simulink subsystem "Stewart_Platform"  (R2019b)
settings: Solver=VariableStepAuto  StartTime=0.0  StopTime=10.0  RelTol=1e-3
settings Model: Creator=thomas  LastModifiedBy=thomas

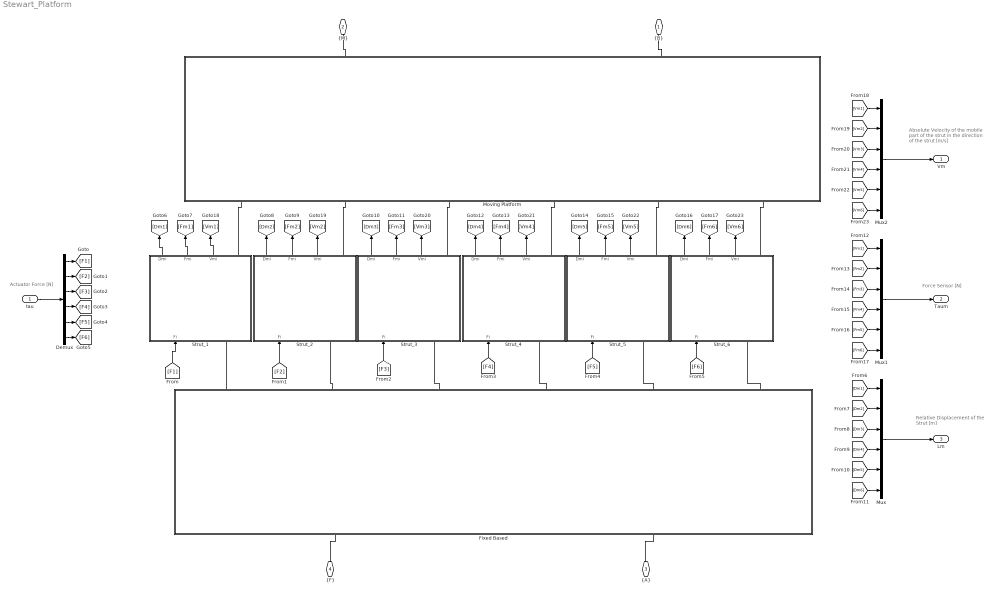
== system Stewart_Platform ==
  note: Force Sensor [N]
  note: Relative Displacement
      | of the Strut [m]
  note: Absolute Velocity of the
      | mobile part of the strut in
      | the direction of the strut [m/s]
  note: Actuator Force [N]
  tau : Inport
  Demux : Demux  Outputs=6
  Fixed Based : Subsystem  ReferencedSubsystem=Fixed_Based
  Moving Platform : Subsystem  ReferencedSubsystem=Mobile_Platform
  Mux : Mux  Inputs=6
  Mux1 : Mux  Inputs=6
  Mux2 : Mux  Inputs=6
  Strut_1 : Subsystem
      mask init:
      | i=1;
  Strut_2 : Subsystem
      mask init:
      | i=2;
  Strut_3 : Subsystem
      mask init:
      | i=3;
  Strut_4 : Subsystem
      mask init:
      | i=4;
  Strut_5 : Subsystem
      mask init:
      | i=5;
  Strut_6 : Subsystem
      mask init:
      | i=6;
  "{B}" : PMIOPort  Side=Right
  "{M}" : PMIOPort  Port=2  Side=Right
  "{A}" : PMIOPort  Port=3  Side=Left
  "{F}" : PMIOPort  Port=4  Side=Left
  Vm : Outport
  Taum : Outport  Port=2
  Lm : Outport  Port=3
  wires:
  [Vm3] -> Mux2/3
  [F3] -> Strut_3/1(Fi)
  [F4] -> Strut_4/1(Fi)
  Strut_5/1(Dmi) -> [Dm5]
  [F1] -> Strut_1/1(Fi)
  Strut_1/2(Fmi) -> [Fm1]
  Demux/5 -> [F5]
  Demux/1 -> [F1]
  Demux/6 -> [F6]
  [Fm2] -> Mux1/2
  Strut_3/1(Dmi) -> [Dm3]
  Demux/3 -> [F3]
  [Fm4] -> Mux1/4
  [Vm2] -> Mux2/2
  [Dm4] -> Mux/4
  Strut_2/1(Dmi) -> [Dm2]
  Strut_6/2(Fmi) -> [Fm6]
  [Vm5] -> Mux2/5
  Strut_1/3(Vmi) -> [Vm1]
  Mux1/1 -> Taum/1
  [Vm1] -> Mux2/1
  Demux/2 -> [F2]
  Mux/1 -> Lm/1
  Strut_6/1(Dmi) -> [Dm6]
  [Dm5] -> Mux/5
  Strut_2/3(Vmi) -> [Vm2]
  [F2] -> Strut_2/1(Fi)
  [Fm6] -> Mux1/6
  Strut_4/1(Dmi) -> [Dm4]
  [Dm2] -> Mux/2
  Strut_6/3(Vmi) -> [Vm6]
  [F5] -> Strut_5/1(Fi)
  [Vm6] -> Mux2/6
  [Fm5] -> Mux1/5
  Strut_3/3(Vmi) -> [Vm3]
  Strut_5/2(Fmi) -> [Fm5]
  Strut_4/2(Fmi) -> [Fm4]
  Strut_5/3(Vmi) -> [Vm5]
  [Vm4] -> Mux2/4
  [F6] -> Strut_6/1(Fi)
  [Fm3] -> Mux1/3
  Mux2/1 -> Vm/1
  [Dm3] -> Mux/3
  tau/1 -> Demux/1
  Strut_3/2(Fmi) -> [Fm3]
  Strut_1/1(Dmi) -> [Dm1]
  Demux/4 -> [F4]
  Strut_2/2(Fmi) -> [Fm2]
  [Dm6] -> Mux/6
  [Fm1] -> Mux1/1
  [Dm1] -> Mux/1
  Strut_4/3(Vmi) -> [Vm4]
  connections:
  Fixed Based/RConn5 -- Strut_5/LConn1
  Fixed Based/RConn1 -- Strut_1/LConn1
  Moving Platform/LConn5 -- Strut_5/RConn1
  Fixed Based/RConn4 -- Strut_4/LConn1
  Fixed Based/RConn3 -- Strut_3/LConn1
  Moving Platform/LConn2 -- Strut_2/RConn1
  Fixed Based/LConn2 -- "{A}"/RConn1
  "{B}"/RConn1 -- Moving Platform/RConn2
  "{F}"/RConn1 -- Fixed Based/LConn1
  Moving Platform/RConn1 -- "{M}"/RConn1
  Fixed Based/RConn6 -- Strut_6/LConn1
  Fixed Based/RConn2 -- Strut_2/LConn1
  Moving Platform/LConn4 -- Strut_4/RConn1
  Moving Platform/LConn6 -- Strut_6/RConn1
  Strut_1/RConn1 -- Moving Platform/LConn1
  Moving Platform/LConn3 -- Strut_3/RConn1

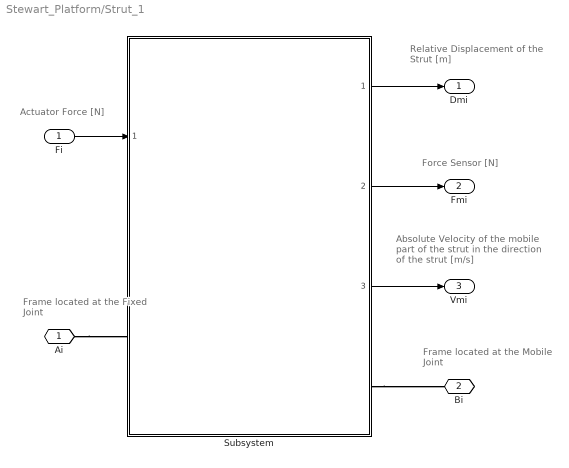
== system Stewart_Platform/Strut_1 ==
  note: Frame located at
      | the Mobile Joint
  note: Actuator Force [N]
  note: Frame located at
      | the Fixed Joint
  note: Force Sensor [N]
  note: Relative Displacement
      | of the Strut [m]
  note: Absolute Velocity of the
      | mobile part of the strut in
      | the direction of the strut [m/s]
  Fi : Inport
  Subsystem : Subsystem  VariantControl=with_sensors  ReferencedSubsystem=stewart_strut
  Ai : PMIOPort  Side=Left
  Bi : PMIOPort  Port=2  Side=Right
  Dmi : Outport
  Fmi : Outport  Port=2
  Vmi : Outport  Port=3
  wires:
  Fi/1 -> Subsystem/1
  Subsystem/3 -> Vmi/1
  Subsystem/2 -> Fmi/1
  Subsystem/1 -> Dmi/1
  connections:
  Subsystem/RConn1 -- Bi/RConn1
  Ai/RConn1 -- Subsystem/LConn1

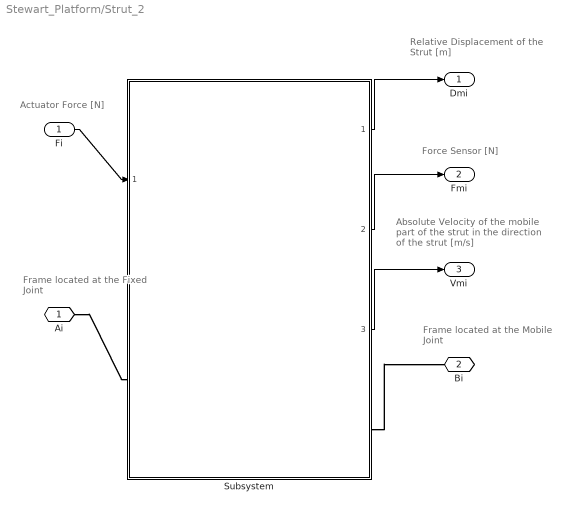
== system Stewart_Platform/Strut_2 ==
  note: Absolute Velocity of the
      | mobile part of the strut in
      | the direction of the strut [m/s]
  note: Relative Displacement
      | of the Strut [m]
  note: Force Sensor [N]
  note: Frame located at
      | the Fixed Joint
  note: Actuator Force [N]
  note: Frame located at
      | the Mobile Joint
  Fi : Inport
  Subsystem : Subsystem  VariantControl=with_sensors  ReferencedSubsystem=stewart_strut
  Ai : PMIOPort  Side=Left
  Bi : PMIOPort  Port=2  Side=Right
  Dmi : Outport
  Fmi : Outport  Port=2
  Vmi : Outport  Port=3
  wires:
  Subsystem/1 -> Dmi/1
  Subsystem/2 -> Fmi/1
  Subsystem/3 -> Vmi/1
  Fi/1 -> Subsystem/1
  connections:
  Ai/RConn1 -- Subsystem/LConn1
  Subsystem/RConn1 -- Bi/RConn1

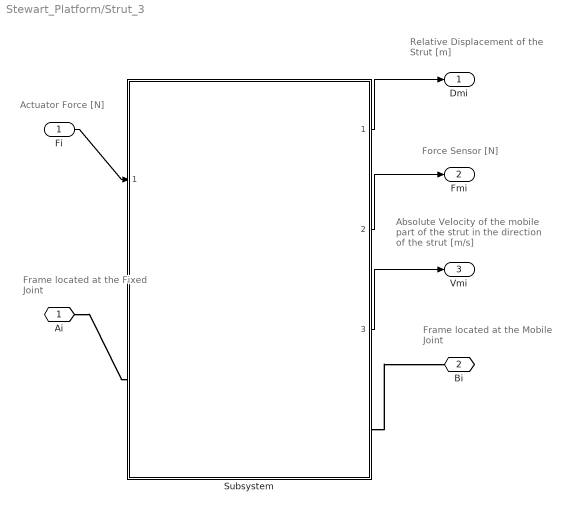
== system Stewart_Platform/Strut_3 ==
  note: Frame located at
      | the Mobile Joint
  note: Actuator Force [N]
  note: Frame located at
      | the Fixed Joint
  note: Force Sensor [N]
  note: Relative Displacement
      | of the Strut [m]
  note: Absolute Velocity of the
      | mobile part of the strut in
      | the direction of the strut [m/s]
  Fi : Inport
  Subsystem : Subsystem  VariantControl=with_sensors  ReferencedSubsystem=stewart_strut
  Ai : PMIOPort  Side=Left
  Bi : PMIOPort  Port=2  Side=Right
  Dmi : Outport
  Fmi : Outport  Port=2
  Vmi : Outport  Port=3
  wires:
  Fi/1 -> Subsystem/1
  Subsystem/3 -> Vmi/1
  Subsystem/2 -> Fmi/1
  Subsystem/1 -> Dmi/1
  connections:
  Subsystem/RConn1 -- Bi/RConn1
  Ai/RConn1 -- Subsystem/LConn1

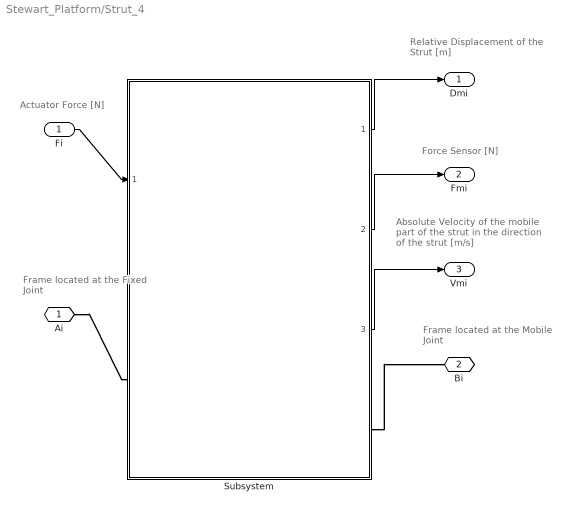
== system Stewart_Platform/Strut_4 ==
  note: Absolute Velocity of the
      | mobile part of the strut in
      | the direction of the strut [m/s]
  note: Relative Displacement
      | of the Strut [m]
  note: Force Sensor [N]
  note: Frame located at
      | the Fixed Joint
  note: Actuator Force [N]
  note: Frame located at
      | the Mobile Joint
  Fi : Inport
  Subsystem : Subsystem  VariantControl=with_sensors  ReferencedSubsystem=stewart_strut
  Ai : PMIOPort  Side=Left
  Bi : PMIOPort  Port=2  Side=Right
  Dmi : Outport
  Fmi : Outport  Port=2
  Vmi : Outport  Port=3
  wires:
  Subsystem/1 -> Dmi/1
  Subsystem/2 -> Fmi/1
  Subsystem/3 -> Vmi/1
  Fi/1 -> Subsystem/1
  connections:
  Ai/RConn1 -- Subsystem/LConn1
  Subsystem/RConn1 -- Bi/RConn1

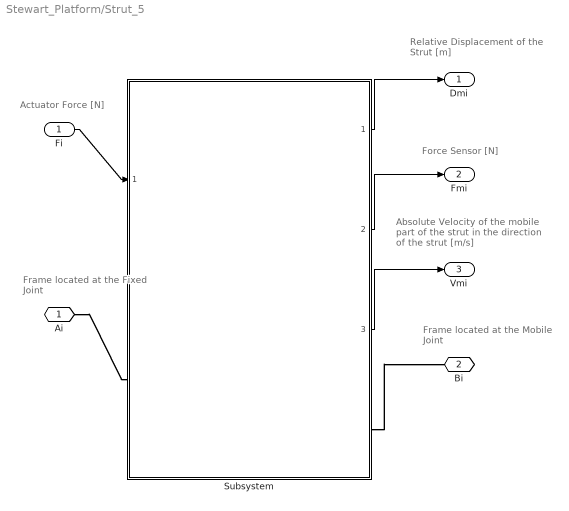
== system Stewart_Platform/Strut_5 ==
  note: Frame located at
      | the Mobile Joint
  note: Actuator Force [N]
  note: Frame located at
      | the Fixed Joint
  note: Force Sensor [N]
  note: Relative Displacement
      | of the Strut [m]
  note: Absolute Velocity of the
      | mobile part of the strut in
      | the direction of the strut [m/s]
  Fi : Inport
  Subsystem : Subsystem  VariantControl=with_sensors  ReferencedSubsystem=stewart_strut
  Ai : PMIOPort  Side=Left
  Bi : PMIOPort  Port=2  Side=Right
  Dmi : Outport
  Fmi : Outport  Port=2
  Vmi : Outport  Port=3
  wires:
  Fi/1 -> Subsystem/1
  Subsystem/3 -> Vmi/1
  Subsystem/2 -> Fmi/1
  Subsystem/1 -> Dmi/1
  connections:
  Subsystem/RConn1 -- Bi/RConn1
  Ai/RConn1 -- Subsystem/LConn1

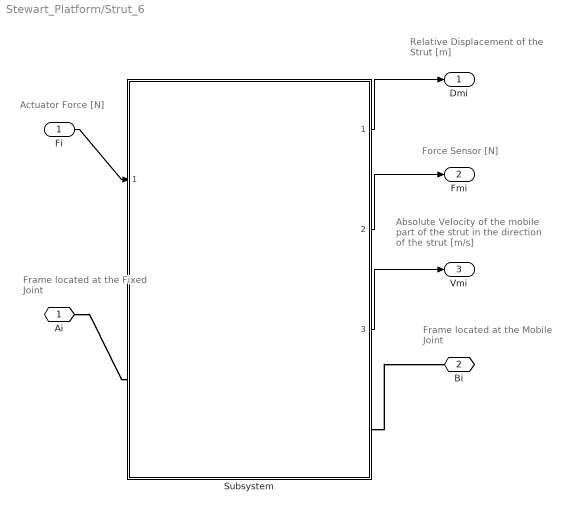
== system Stewart_Platform/Strut_6 ==
  note: Absolute Velocity of the
      | mobile part of the strut in
      | the direction of the strut [m/s]
  note: Relative Displacement
      | of the Strut [m]
  note: Force Sensor [N]
  note: Frame located at
      | the Fixed Joint
  note: Actuator Force [N]
  note: Frame located at
      | the Mobile Joint
  Fi : Inport
  Subsystem : Subsystem  VariantControl=with_sensors  ReferencedSubsystem=stewart_strut
  Ai : PMIOPort  Side=Left
  Bi : PMIOPort  Port=2  Side=Right
  Dmi : Outport
  Fmi : Outport  Port=2
  Vmi : Outport  Port=3
  wires:
  Subsystem/1 -> Dmi/1
  Subsystem/2 -> Fmi/1
  Subsystem/3 -> Vmi/1
  Fi/1 -> Subsystem/1
  connections:
  Ai/RConn1 -- Subsystem/LConn1
  Subsystem/RConn1 -- Bi/RConn1
